simulink model "SimulationContinueClampingMCC"  (R2017b)
settings: Solver=VariableStepAuto  StartTime=0.0  StopTime=Tf  MaxStep=1e-4  RelTol=1e-3
values from neighbouring files (symbols this model uses):
  C0 = 0.0    (= 0)    [DCMotorParameters.m]    (also in DonneesMCC.m)
  Cl = .0    (= 0)    [DCMotorParameters.m]    (also in DonneesMCC.m)
  F = 0.0001    [DCMotorParameters.m]    (also in DonneesMCC.m)
  Imax = Inom    (= 5)    [DCMotorParameters.m]    (also in DonneesMCC.m)
  Imin = -Inom    (= -5)    [DCMotorParameters.m]    (also in DonneesMCC.m)
  J = 2.20e-4    (= 0.00022)    [DCMotorParameters.m]    (also in DonneesMCC.m)
  Kelec = place(Ae,Be,Elec_desired_poles)    [DCMotorParameters.m]    (also in DonneesMCC.m = -place(Ae,Be,Pole_elec_desiree))
  Kmeca = place(Am,Bm,Pole_meca_desiree)    [DCMotorParameters.m]    (also in DonneesMCC.m)
  Kphi = 0.061    [DCMotorParameters.m]    (also in DonneesMCC.m)
  L = 2.7e-3    (= 0.0027)    [DCMotorParameters.m]    (also in DonneesMCC.m)
  omref = 200    [DCMotorParameters.m]    (also in DonneesMCC.m)
  R = 1.22    [DCMotorParameters.m]    (also in DonneesMCC.m)
  Ts = 1e-4    (= 0.0001)    [DCMotorParameters.m]    (also in DonneesMCC.m)
  Vmax = Vdc    (= 24)    [DCMotorParameters.m]    (also in DonneesMCC.m)
  Vmin = -Vdc    (= -24)    [DCMotorParameters.m]    (also in DonneesMCC.m)
settings Model: Creator=romaindelpoux  LastModifiedBy=rdelpoux
settings SolverCC: ZeroCrossControl=DisableAll

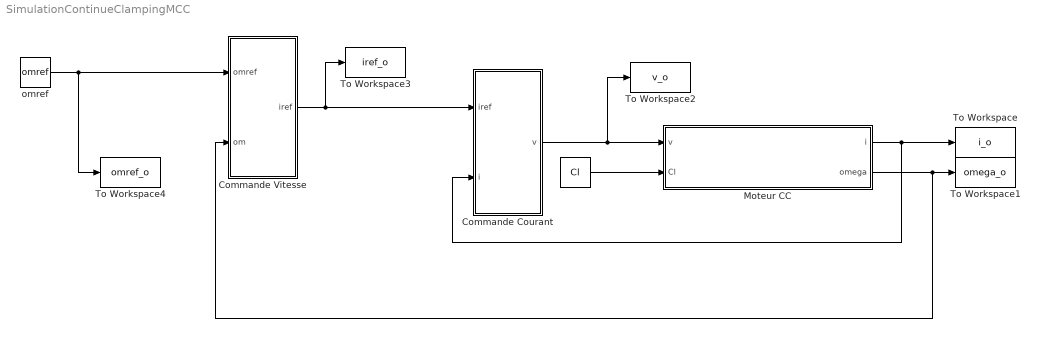
== system SimulationContinueClampingMCC ==
  " " : Constant  Value=Cl
  Commande Courant : Subsystem
  Commande Vitesse : Subsystem
  Moteur CC : Subsystem
  To Workspace : ToWorkspace  VariableName=i_o  SaveFormat=Timeseries  SampleTime=-1
  To Workspace1 : ToWorkspace  VariableName=omega_o  SaveFormat=Timeseries  SampleTime=-1
  To Workspace2 : ToWorkspace  VariableName=v_o  SaveFormat=Timeseries  SampleTime=-1
  To Workspace3 : ToWorkspace  VariableName=iref_o  SaveFormat=Timeseries  SampleTime=-1
  To Workspace4 : ToWorkspace  VariableName=omref_o  SaveFormat=Timeseries  SampleTime=-1
  omref : Constant  Value=omref
  wires:
  Commande Courant/1(v) -> To Workspace2/1, Moteur CC/1(v)
  Moteur CC/2(omega) -> Commande Vitesse/2(om), To Workspace1/1
  Moteur CC/1(i) -> Commande Courant/2(i), To Workspace/1
  omref/1 -> To Workspace4/1, Commande Vitesse/1(omref)
  Commande Vitesse/1(iref) -> Commande Courant/1(iref), To Workspace3/1
  " "/1 -> Moteur CC/2(Cl)

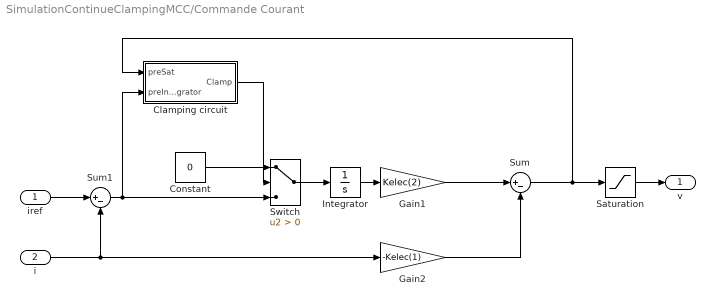
== system SimulationContinueClampingMCC/Commande Courant ==
  iref : Inport
  i : Inport  Port=2
  Clamping circuit : Subsystem
  Constant : Constant  Value=0
  Gain1 : Gain  Gain=Kelec(2)
  Gain2 : Gain  Gain=-Kelec(1)
  Integrator : Integrator
  Saturation : Saturate  UpperLimit=Vmax  LowerLimit=Vmin
  Sum : Sum  Inputs=|+-
  Sum1 : Sum  Inputs=|+-
  Switch : Switch  Criteria=u2 > Threshold  InputSameDT=on
  v : Outport
  wires:
  iref/1 -> Sum1/1
  i/1 -> Gain2/1, Sum1/2
  Integrator/1 -> Gain1/1
  Gain1/1 -> Sum/1
  Gain2/1 -> Sum/2
  Constant/1 -> Switch/1
  Sum/1 -> Saturation/1, Clamping circuit/1(preSat)
  Sum1/1 -> Switch/3, Clamping circuit/2(preIntegrator)
  Clamping circuit/1(Clamp) -> Switch/2
  Saturation/1 -> v/1
  Switch/1 -> Integrator/1

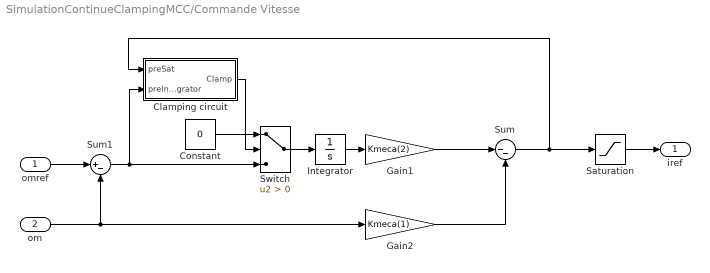
== system SimulationContinueClampingMCC/Commande Vitesse ==
  omref : Inport
  om : Inport  Port=2
  Clamping circuit : Subsystem
  Constant : Constant  Value=0
  Gain1 : Gain  Gain=Kmeca(2)
  Gain2 : Gain  Gain=Kmeca(1)
  Integrator : Integrator
  Saturation : Saturate  UpperLimit=Imax  LowerLimit=Imin
  Sum : Sum  Inputs=|--
  Sum1 : Sum  Inputs=|+-
  Switch : Switch  Criteria=u2 > Threshold  InputSameDT=on
  iref : Outport
  wires:
  Gain1/1 -> Sum/1
  Integrator/1 -> Gain1/1
  omref/1 -> Sum1/1
  Gain2/1 -> Sum/2
  om/1 -> Gain2/1, Sum1/2
  Sum/1 -> Clamping circuit/1(preSat), Saturation/1
  Saturation/1 -> iref/1
  Switch/1 -> Integrator/1
  Sum1/1 -> Switch/3, Clamping circuit/2(preIntegrator)
  Clamping circuit/1(Clamp) -> Switch/2
  Constant/1 -> Switch/1

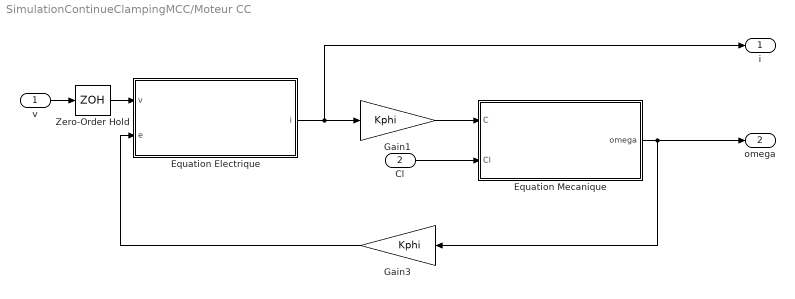
== system SimulationContinueClampingMCC/Moteur CC ==
  v : Inport
  Cl : Inport  Port=2
  Equation Electrique : Subsystem
  Equation Mecanique : Subsystem
  Gain1 : Gain  Gain=Kphi
  "Gain3  " : Gain  Gain=Kphi
  Zero-Order Hold : ZeroOrderHold  SampleTime=Ts
  i : Outport
  omega : Outport  Port=2
  wires:
  v/1 -> Zero-Order Hold/1
  "Gain3  "/1 -> Equation Electrique/2(e)
  Gain1/1 -> Equation Mecanique/1(C)
  Cl/1 -> Equation Mecanique/2(Cl)
  Zero-Order Hold/1 -> Equation Electrique/1(v)
  Equation Electrique/1(i) -> i/1, Gain1/1
  Equation Mecanique/1(omega) -> omega/1, "Gain3  "/1

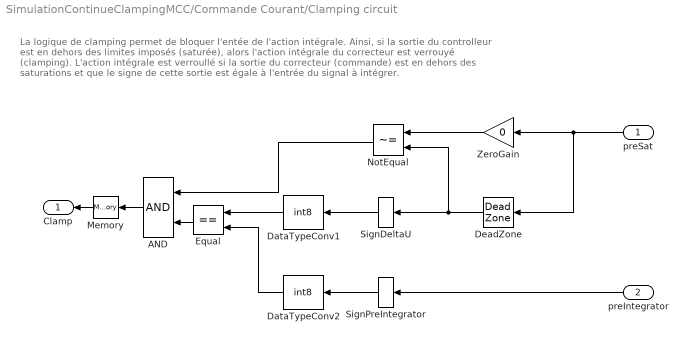
== system SimulationContinueClampingMCC/Commande Courant/Clamping circuit ==
  note: La logique de clamping permet de bloquer l'entée de l'action intégrale.
      | Ainsi, si la sortie du controlleur est en dehors des limites imposés (saturée), alors l'action intégrale du correcteur est verrouyé (clamping).
      | L'action intégrale est verroullé si la sortie du correcteur (commande) est en dehors des saturations et que le signe de cette sortie est égale
      | à l'entrée du signal à intégrer.
  preSat : Inport  DisableCoverage=on
  preIntegrator : Inport  DisableCoverage=on  Port=2
  AND : Logic  DisableCoverage=on
  DataTypeConv1 : DataTypeConversion  DisableCoverage=on  OutDataTypeStr=int8  SaturateOnIntegerOverflow=on  RndMeth=Zero  LockScale=on
  DataTypeConv2 : DataTypeConversion  DisableCoverage=on  OutDataTypeStr=int8
  DeadZone : DeadZone  DisableCoverage=on  LowerValue=Vmin  UpperValue=Vmax
  Equal : RelationalOperator  DisableCoverage=on  Operator===  RndMeth=Nearest  InputSameDT=on
  Memory : Memory  DisableCoverage=on
  NotEqual : RelationalOperator  DisableCoverage=on  Operator=~=  RndMeth=Nearest  InputSameDT=on
  SignDeltaU : Signum  DisableCoverage=on
  SignPreIntegrator : Signum  DisableCoverage=on
  ZeroGain : Gain  DisableCoverage=on  Gain=0  SaturateOnIntegerOverflow=on  OutDataTypeStr=Inherit: Same as input  ParamDataTypeStr=Inherit: Same as input
  Clamp : Outport  DisableCoverage=on
  wires:
  preSat/1 -> ZeroGain/1, DeadZone/1
  preIntegrator/1 -> SignPreIntegrator/1
  ZeroGain/1 -> NotEqual/1
  DeadZone/1 -> NotEqual/2, SignDeltaU/1
  SignDeltaU/1 -> DataTypeConv1/1
  DataTypeConv1/1 -> Equal/1
  SignPreIntegrator/1 -> DataTypeConv2/1
  DataTypeConv2/1 -> Equal/2
  NotEqual/1 -> AND/1
  Equal/1 -> AND/2
  AND/1 -> Memory/1
  Memory/1 -> Clamp/1

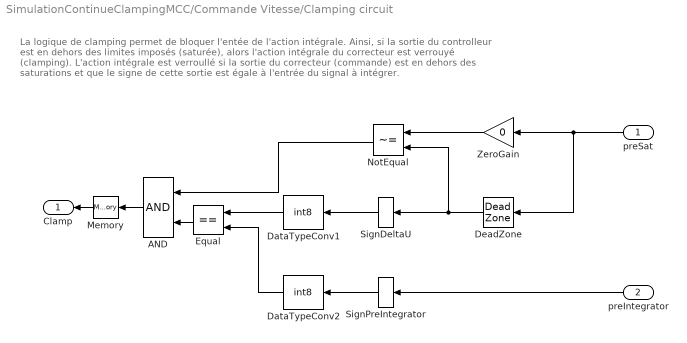
== system SimulationContinueClampingMCC/Commande Vitesse/Clamping circuit ==
  note: La logique de clamping permet de bloquer l'entée de l'action intégrale.
      | Ainsi, si la sortie du controlleur est en dehors des limites imposés (saturée), alors l'action intégrale du correcteur est verrouyé (clamping).
      | L'action intégrale est verroullé si la sortie du correcteur (commande) est en dehors des saturations et que le signe de cette sortie est égale
      | à l'entrée du signal à intégrer.
  preSat : Inport  DisableCoverage=on
  preIntegrator : Inport  DisableCoverage=on  Port=2
  AND : Logic  DisableCoverage=on
  DataTypeConv1 : DataTypeConversion  DisableCoverage=on  OutDataTypeStr=int8  SaturateOnIntegerOverflow=on  RndMeth=Zero  LockScale=on
  DataTypeConv2 : DataTypeConversion  DisableCoverage=on  OutDataTypeStr=int8
  DeadZone : DeadZone  DisableCoverage=on  LowerValue=Imin  UpperValue=Imax
  Equal : RelationalOperator  DisableCoverage=on  Operator===  RndMeth=Nearest  InputSameDT=on
  Memory : Memory  DisableCoverage=on
  NotEqual : RelationalOperator  DisableCoverage=on  Operator=~=  RndMeth=Nearest  InputSameDT=on
  SignDeltaU : Signum  DisableCoverage=on
  SignPreIntegrator : Signum  DisableCoverage=on
  ZeroGain : Gain  DisableCoverage=on  Gain=0  SaturateOnIntegerOverflow=on  OutDataTypeStr=Inherit: Same as input  ParamDataTypeStr=Inherit: Same as input
  Clamp : Outport  DisableCoverage=on
  wires:
  preSat/1 -> ZeroGain/1, DeadZone/1
  preIntegrator/1 -> SignPreIntegrator/1
  ZeroGain/1 -> NotEqual/1
  DeadZone/1 -> NotEqual/2, SignDeltaU/1
  SignDeltaU/1 -> DataTypeConv1/1
  DataTypeConv1/1 -> Equal/1
  SignPreIntegrator/1 -> DataTypeConv2/1
  DataTypeConv2/1 -> Equal/2
  NotEqual/1 -> AND/1
  Equal/1 -> AND/2
  AND/1 -> Memory/1
  Memory/1 -> Clamp/1

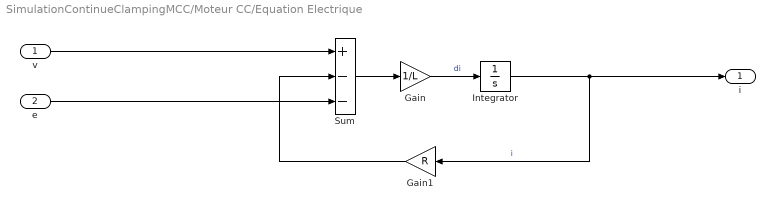
== system SimulationContinueClampingMCC/Moteur CC/Equation Electrique ==
  v : Inport
  e : Inport  Port=2
  Gain : Gain  Gain=1/L
  Gain1 : Gain  Gain=R
  Integrator : Integrator
  Sum : Sum  Inputs=+--
  i : Outport
  wires:
  Gain1/1 -> Sum/2
  Sum/1 -> Gain/1
  Integrator/1 -> i/1, Gain1/1  "i"
  Gain/1 -> Integrator/1  "di"
  v/1 -> Sum/1
  e/1 -> Sum/3

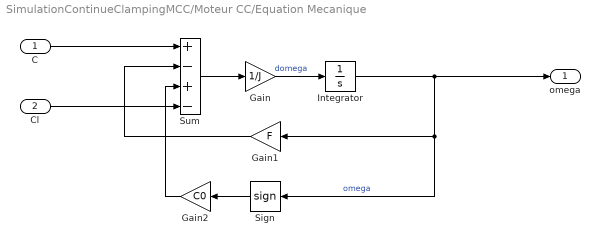
== system SimulationContinueClampingMCC/Moteur CC/Equation Mecanique ==
  C : Inport
  Cl : Inport  Port=2
  Gain : Gain  Gain=1/J
  Gain1 : Gain  Gain=F
  Gain2 : Gain  Gain=C0
  Integrator : Integrator
  Sign : Signum
  Sum : Sum  Inputs=+-+-
  omega : Outport
  wires:
  Gain/1 -> Integrator/1  "domega"
  Integrator/1 -> Sign/1, Gain1/1, omega/1  "omega"
  Sum/1 -> Gain/1
  Gain1/1 -> Sum/2
  Sign/1 -> Gain2/1
  Gain2/1 -> Sum/3
  C/1 -> Sum/1
  Cl/1 -> Sum/4
